simulink model "gnc_simplified"  (R2025b)
settings: Solver=ode2  StartTime=0.0  StopTime=inf  FixedStep=1/100  RelTol=1e-3
undefined symbols (not defined in the file or in its folder): DiscIntNeverNeededParam, dspblkCoreblockFVToolHelper, gcbh
libraries: simulink x5, eeGeneralControl x5
(part 4 of 4)

== matlab function gnc_simplified/INDI/Rates to surfaces&brakes/Diff and Filter IMU/fromRPAS/Subsystem/MATLAB Function8 ==
  data: omega input single; zeta input single; filt_num output single; filt_den output single
function [filt_num,filt_den]  = tbv(omega, zeta)

T = single(0.01);
w = omega;
z = zeta;

scale = T^2*w^2+4*T*w*z+4;

filt_num = [T^2*w^2, 2*T^2*w^2, T^2*w^2]/scale;
filt_den = [T^2*w^2+4*T*w*z+4 2*T^2*w^2-8 T^2*w^2-4*T*w*z+4]/scale;

== matlab function gnc_simplified/INDI/Rates to surfaces&brakes/Diff and Filter IMU/fromRPAS/Subsystem/MATLAB Function9 ==
  data: omega input single; zeta input single; filt_num output single; filt_den output single
function [filt_num,filt_den]  = tbv(omega, zeta)

T = single(0.01);
w = omega;
z = zeta;

scale = T^2*w^2+4*T*w*z+4;

filt_num = [T^2*w^2, 2*T^2*w^2, T^2*w^2]/scale;
filt_den = [T^2*w^2+4*T*w*z+4 2*T^2*w^2-8 T^2*w^2-4*T*w*z+4]/scale;

== matlab function gnc_simplified/Modal/limit control output ==
  data: u input; y output single
function y = control_output_sat(u)

y = zeros(size(u),'single');
y(:) = min(max(u(:),-1),1);

end

== matlab function gnc_simplified/ATOL_Guidance ==
  settings: updateMethod=DISCRETE
  data: AP_mode input uint8; params input Bus: IFRCG_Bus_Params_Gnc; guidance_out output Bus: IFRCG_Bus_GuidanceCmd
function guidance_out  = Guidance(AP_mode,params)

%% Instantiate output signals
thetaCmd = single(0);
psiCmd   = single(0);
phiCmd   = single(0);
gammaCmd  = single(0);
chiCmd   = single(0);
vCmd      = single(0);

%% Guidance

switch AP_mode
    case 1 % Test controls on ground
        phiCmd = single(0);
        thetaCmd = single(0);
        psiCmd = single(0);
    case 2 %steady_state
        phiCmd = single(0); %wings level
        gammaCmd = params.Ifr_Gnc.GU_GAMMA_CMD*pi/180;
        vCmd = params.Ifr_Gnc.GU_V_CMD;
    otherwise %(case 3) track following
        gammaCmd = params.Ifr_Gnc.GU_GAMMA_CMD*pi/180;
        chi = params.Ifr_Gnc.GU_CHI_CMD*pi/180;
        chiCmd = mod((chi+pi),2*pi)-pi;
        vCmd = params.Ifr_Gnc.GU_V_CMD;
end

% Summarize command values
guidance_out.roll_lim = single(45*pi/180);
guidance_out.act_cmd = zeros(6,1,'single');
guidance_out.rte_cmd = zeros(3,1,'single');
guidance_out.att_cmd = [single(0);thetaCmd;single(0);psiCmd;phiCmd];
guidance_out.trk_cmd = [gammaCmd;chiCmd;vCmd];

end
